simulink model "tcs_VHF_model_free"  (R2022b)
settings: Solver=FixedStepAuto  StartTime=0.0  StopTime=6.5  RelTol=1e-3
PreLoadFcn:
  | run('control_bus.m')
model workspace (MAT data in the model file):
  Tmax = 1000
  re = 0.284
libraries: simulink x4, Solver_SF x1
CloseFcn:
  | clear control_info_bus
settings Model: Creator=henri  LastModifiedBy=Henrique Mesquita
settings DebuggingCC: UnconnectedInputMsg=warning  UnconnectedOutputMsg=warning  UnconnectedLineMsg=warning
settings ModelReferenceCC: EnableRefExpFcnMdlSchedulingChecks=on
settings RTWCC: DLArmComputeVersion=19.05

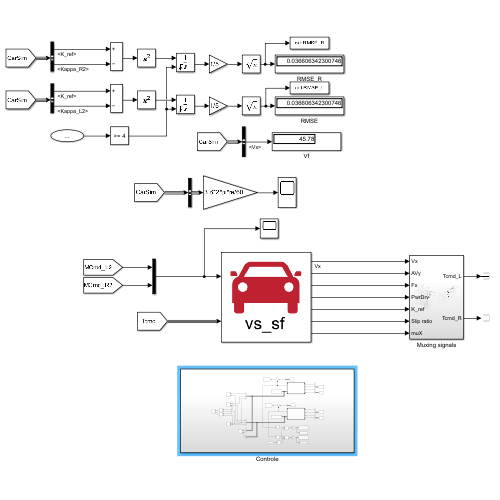
[thumbnail: Simulink's stored preview of the top-level diagram]
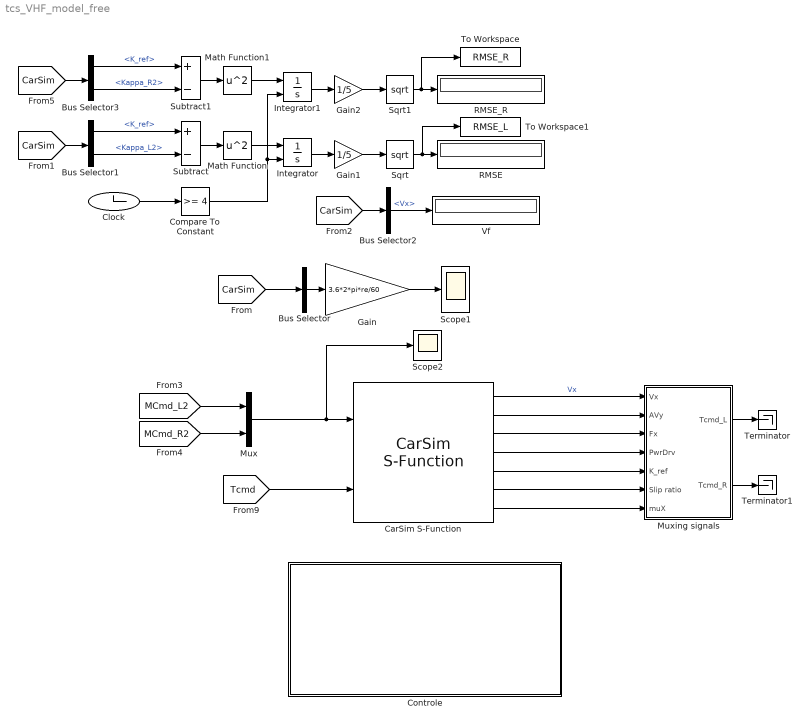
== system tcs_VHF_model_free ==
  Bus Selector : BusSelector  OutputSignals=AVy_L1,AVy_R1,AVy_L2,AVy_R2  OutputAsBus=on
  Bus Selector1 : BusSelector  OutputSignals=K_ref,Kappa_L2
  Bus Selector2 : BusSelector  OutputSignals=Vx
  Bus Selector3 : BusSelector  OutputSignals=K_ref,Kappa_R2
  CarSim S-Function : Solver_SF/CarSim S-Function  Priority=1  SIMFILE=simfile.sim  Run_RTs=off  vs_state_ind=Run  StopMode_ind=Vehicle Model
  Clock : Clock
  Compare To Constant : simulink/Logic and Bit Operations/Compare To Constant  relop=>=  const=4  OutDataTypeStr=boolean
  Controle : Subsystem
  Gain : Gain  Gain=3.6*2*pi*re/60
  Gain1 : Gain  Gain=1/5
  Gain2 : Gain  Gain=1/5
  Integrator : Integrator  ExternalReset=rising
  Integrator1 : Integrator  ExternalReset=rising
  Math Function : Math  Operator=square
  Math Function1 : Math  Operator=square
  Mux : Mux  Inputs=2
  Muxing signals : Subsystem
  RMSE : Display
  RMSE_R : Display
  Scope1 : Scope
  Scope2 : Scope
  Sqrt : Sqrt
  Sqrt1 : Sqrt
  Subtract : Sum  Inputs=+-
  Subtract1 : Sum  Inputs=+-
  Terminator : Terminator
  Terminator1 : Terminator
  To Workspace : ToWorkspace  VariableName=RMSE_R  SampleTime=-1
      settings: MaxDataPoints=1  Save2DSignal=2-D array (concatenate along first dimension)
  To Workspace1 : ToWorkspace  VariableName=RMSE_L  SampleTime=-1
      settings: MaxDataPoints=1  Save2DSignal=2-D array (concatenate along first dimension)
  Vf : Display
  wires:
  Mux/1 -> Scope2/1, CarSim S-Function/1
  [CarSim] -> Bus Selector/1
  Bus Selector/1 -> Gain/1
  [MCmd_R2] -> Mux/2
  [MCmd_L2] -> Mux/1
  [Tcmd] -> CarSim S-Function/2
  CarSim S-Function/1 -> Muxing signals/1(Vx)  "Vx"
  CarSim S-Function/2 -> Muxing signals/2(AVy)
  CarSim S-Function/3 -> Muxing signals/3(Fx)
  CarSim S-Function/4 -> Muxing signals/4(PwrDrv)
  CarSim S-Function/6 -> Muxing signals/6(Slip ratio)
  Muxing signals/2(Tcmd_R) -> Terminator1/1
  Muxing signals/1(Tcmd_L) -> Terminator/1
  CarSim S-Function/5 -> Muxing signals/5(K_ref)
  CarSim S-Function/7 -> Muxing signals/7(muX)
  Gain/1 -> Scope1/1
  [CarSim] -> Bus Selector1/1
  Bus Selector1/2 -> Subtract/2  "<Kappa_L2>"
  Bus Selector1/1 -> Subtract/1  "<K_ref>"
  Integrator/1 -> Gain1/1
  Gain1/1 -> Sqrt/1
  Subtract/1 -> Math Function/1
  Math Function/1 -> Integrator/1
  Sqrt/1 -> To Workspace1/1, RMSE/1
  [CarSim] -> Bus Selector2/1
  Bus Selector2/1 -> Vf/1  "<Vx>"
  Sqrt1/1 -> To Workspace/1, RMSE_R/1
  Integrator1/1 -> Gain2/1
  Gain2/1 -> Sqrt1/1
  Subtract1/1 -> Math Function1/1
  Bus Selector3/1 -> Subtract1/1  "<K_ref>"
  [CarSim] -> Bus Selector3/1
  Math Function1/1 -> Integrator1/1
  Bus Selector3/2 -> Subtract1/2  "<Kappa_R2>"
  Clock/1 -> Compare To Constant/1
  Compare To Constant/1 -> Integrator/2, Integrator1/2

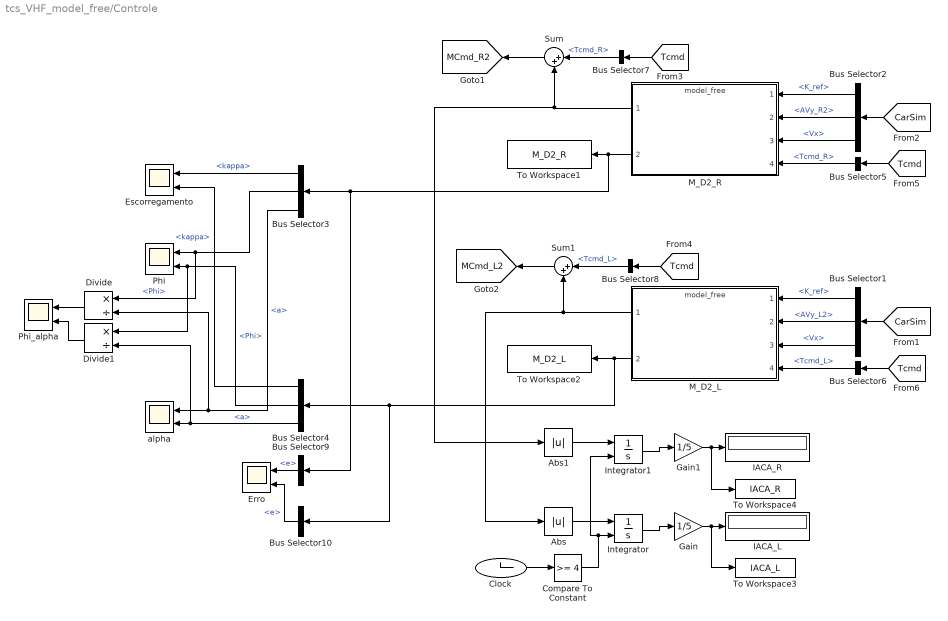
== system tcs_VHF_model_free/Controle ==
  Abs : Abs  SaturateOnIntegerOverflow=off
  Abs1 : Abs  SaturateOnIntegerOverflow=off
  Bus Selector1 : BusSelector  OutputSignals=K_ref,AVy_L2,Vx
  Bus Selector10 : BusSelector  OutputSignals=e
  Bus Selector2 : BusSelector  OutputSignals=K_ref,AVy_R2,Vx
  Bus Selector3 : BusSelector  OutputSignals=kappa,Phi,a
  Bus Selector4 : BusSelector  OutputSignals=kappa,Phi,a
  Bus Selector5 : BusSelector  OutputSignals=Tcmd_R
  Bus Selector6 : BusSelector  OutputSignals=Tcmd_L
  Bus Selector7 : BusSelector  OutputSignals=Tcmd_R
  Bus Selector8 : BusSelector  OutputSignals=Tcmd_L
  Bus Selector9 : BusSelector  OutputSignals=e
  Clock : Clock
  Compare To Constant : simulink/Logic and Bit Operations/Compare To Constant  relop=>=  const=4  OutDataTypeStr=boolean
  Divide : Product  Inputs=*/
  Divide1 : Product  Inputs=*/
  Erro : Scope  NumInputPorts=2
  "Escorregamento " : Scope  NumInputPorts=2
  Gain : Gain  Gain=1/5
  Gain1 : Gain  Gain=1/5
  IACA_L : Display
  IACA_R : Display
  Integrator : Integrator  ExternalReset=rising
  Integrator1 : Integrator  ExternalReset=rising
  M_D2_L : ModelReference  ModelNameDialog=model_free.slx  SimulationMode=Normal  ModelReferenceVersion=4.1
  M_D2_R : ModelReference  ModelNameDialog=model_free.slx  SimulationMode=Normal  ModelReferenceVersion=4.1
  Phi : Scope  NumInputPorts=2
  Phi_alpha : Scope  NumInputPorts=2
  Sum : Sum  Inputs=|++
  Sum1 : Sum  Inputs=|++
  To Workspace1 : ToWorkspace  VariableName=M_D2_R  SaveFormat=Timeseries  SampleTime=-1
  To Workspace2 : ToWorkspace  VariableName=M_D2_L  SaveFormat=Timeseries  SampleTime=-1
  To Workspace3 : ToWorkspace  VariableName=IACA_L  SampleTime=-1
      settings: MaxDataPoints=1  Save2DSignal=2-D array (concatenate along first dimension)
  To Workspace4 : ToWorkspace  VariableName=IACA_R  SampleTime=-1
      settings: MaxDataPoints=1  Save2DSignal=2-D array (concatenate along first dimension)
  alpha : Scope  NumInputPorts=2
  tag scope: MCmd_L2=global, MCmd_R2=global
  wires:
  Bus Selector4/3 -> Divide1/2, alpha/2  "<a>"
  M_D2_L/2 -> To Workspace2/1, Bus Selector10/1, Bus Selector4/1
  M_D2_R/2 -> To Workspace1/1, Bus Selector9/1, Bus Selector3/1
  [CarSim] -> Bus Selector1/1
  Bus Selector1/2 -> M_D2_L/2  "<AVy_L2>"
  Bus Selector2/2 -> M_D2_R/2  "<AVy_R2>"
  Bus Selector1/3 -> M_D2_L/3  "<Vx>"
  [CarSim] -> Bus Selector2/1
  Bus Selector2/3 -> M_D2_R/3  "<Vx>"
  Bus Selector6/1 -> M_D2_L/4  "<Tcmd_L>"
  Bus Selector4/2 -> Divide1/1, Phi/2  "<Phi>"
  Bus Selector3/2 -> Divide/1, Phi/1  "<Phi>"
  Bus Selector4/1 -> "Escorregamento "/2  "<kappa>"
  M_D2_R/1 -> Abs1/1, Sum/2
  Bus Selector3/1 -> "Escorregamento "/1  "<kappa>"
  [Tcmd] -> Bus Selector6/1
  Bus Selector2/1 -> M_D2_R/1  "<K_ref>"
  Bus Selector1/1 -> M_D2_L/1  "<K_ref>"
  [Tcmd] -> Bus Selector5/1
  Bus Selector3/3 -> Divide/2, alpha/1  "<a>"
  Bus Selector5/1 -> M_D2_R/4  "<Tcmd_R>"
  Sum/1 -> [MCmd_R2]
  [Tcmd] -> Bus Selector7/1
  Bus Selector7/1 -> Sum/1  "<Tcmd_R>"
  Bus Selector8/1 -> Sum1/1  "<Tcmd_L>"
  [Tcmd] -> Bus Selector8/1
  M_D2_L/1 -> Abs/1, Sum1/2
  Sum1/1 -> [MCmd_L2]
  Divide/1 -> Phi_alpha/1
  Divide1/1 -> Phi_alpha/2
  Bus Selector9/1 -> Erro/1  "<e>"
  Bus Selector10/1 -> Erro/2  "<e>"
  Abs/1 -> Integrator/1
  Integrator/1 -> Gain/1
  Gain/1 -> To Workspace3/1, IACA_L/1
  Clock/1 -> Compare To Constant/1
  Compare To Constant/1 -> Integrator/2, Integrator1/2
  Abs1/1 -> Integrator1/1
  Gain1/1 -> To Workspace4/1, IACA_R/1
  Integrator1/1 -> Gain1/1

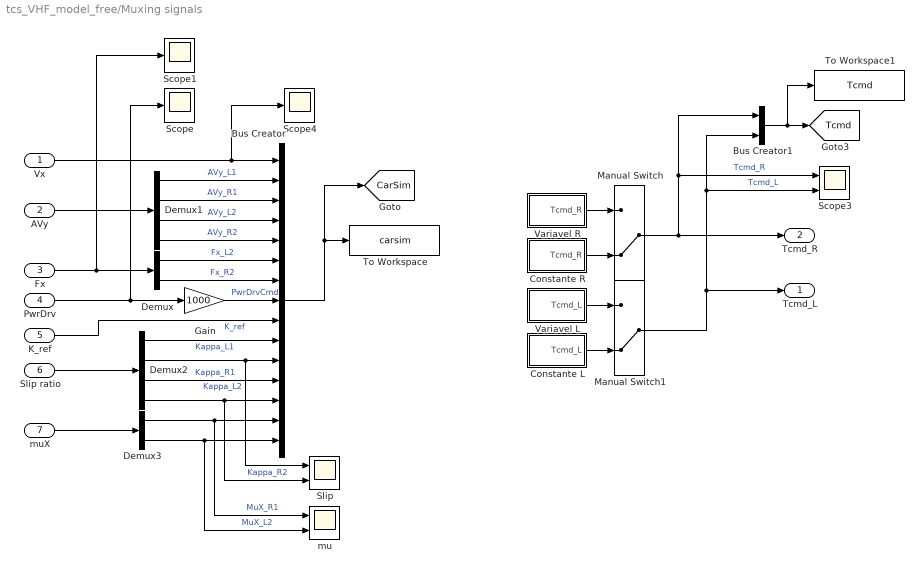
== system tcs_VHF_model_free/Muxing signals ==
  Vx : Inport
  AVy : Inport  Port=2
  Fx : Inport  Port=3
  PwrDrv : Inport  Port=4
  K_ref : Inport  Port=5
  Slip ratio : Inport  Port=6
  muX : Inport  Port=7
  Bus Creator : BusCreator  Inputs=15
  Bus Creator1 : BusCreator  Inputs=2
  Constante L : Subsystem
  Constante R : Subsystem
  Demux : Demux  Outputs=2
  Demux1 : Demux
  Demux2 : Demux
  Demux3 : Demux  Outputs=2
  Gain : Gain  Gain=1000
  Manual Switch : ManualSwitch  CurrentSetting=0
  Manual Switch1 : ManualSwitch  CurrentSetting=0
  Scope : Scope
  Scope1 : Scope
  Scope3 : Scope  NumInputPorts=2
  Scope4 : Scope
  Slip : Scope  NumInputPorts=2
  To Workspace : ToWorkspace  VariableName=carsim  SaveFormat=Timeseries  SampleTime=-1
  To Workspace1 : ToWorkspace  VariableName=Tcmd  SaveFormat=Timeseries  SampleTime=-1
  Variavel L : Subsystem
  Variavel R : Subsystem
  mu : Scope  NumInputPorts=2
  Tcmd_L : Outport
  Tcmd_R : Outport  Port=2
  tag scope: CarSim=global, Tcmd=global
  wires:
  K_ref/1 -> Bus Creator/9  "K_ref"
  Demux1/3 -> Bus Creator/4  "AVy_L2"
  Bus Creator/1 -> [CarSim], To Workspace/1
  Demux/2 -> Bus Creator/7  "Fx_R2"
  Vx/1 -> Scope4/1, Bus Creator/1
  Demux1/1 -> Bus Creator/2  "AVy_L1"
  Demux1/4 -> Bus Creator/5  "AVy_R2"
  PwrDrv/1 -> Gain/1, Scope/1
  Demux/1 -> Bus Creator/6  "Fx_L2"
  Gain/1 -> Bus Creator/8  "PwrDrvCmd"
  Demux1/2 -> Bus Creator/3  "AVy_R1"
  Fx/1 -> Scope1/1, Demux/1
  AVy/1 -> Demux1/1
  Bus Creator1/1 -> To Workspace1/1, [Tcmd]
  Manual Switch/1 -> Bus Creator1/1, Scope3/1, Tcmd_R/1  "Tcmd_R"
  Manual Switch1/1 -> Bus Creator1/2, Scope3/2, Tcmd_L/1  "Tcmd_L"
  Slip ratio/1 -> Demux2/1
  Demux2/1 -> Bus Creator/10  "Kappa_L1"
  Demux2/2 -> Slip/1, Bus Creator/11  "Kappa_L2"
  Demux2/3 -> Bus Creator/12  "Kappa_R1"
  Demux2/4 -> Slip/2, Bus Creator/13  "Kappa_R2"
  Variavel R/1(Tcmd_R) -> Manual Switch/1
  Constante R/1(Tcmd_R) -> Manual Switch/2
  Constante L/1(Tcmd_L) -> Manual Switch1/2
  Variavel L/1(Tcmd_L) -> Manual Switch1/1
  muX/1 -> Demux3/1
  Demux3/1 -> mu/1, Bus Creator/14  "MuX_R1"
  Demux3/2 -> mu/2, Bus Creator/15  "MuX_L2"

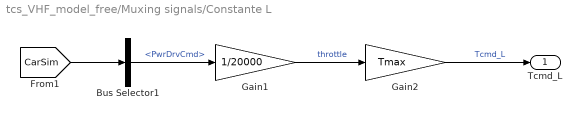
== system tcs_VHF_model_free/Muxing signals/Constante L ==
  Bus Selector1 : BusSelector  OutputSignals=PwrDrvCmd
  Gain1 : Gain  Gain=1/20000
  Gain2 : Gain  Gain=Tmax
  Tcmd_L : Outport
  wires:
  Gain2/1 -> Tcmd_L/1  "Tcmd_L"
  Gain1/1 -> Gain2/1  "throttle"
  [CarSim] -> Bus Selector1/1
  Bus Selector1/1 -> Gain1/1  "<PwrDrvCmd>"

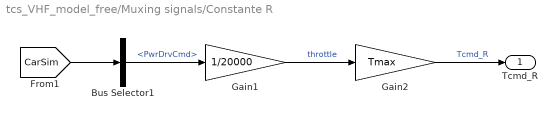
== system tcs_VHF_model_free/Muxing signals/Constante R ==
  Bus Selector1 : BusSelector  OutputSignals=PwrDrvCmd
  Gain1 : Gain  Gain=1/20000
  Gain2 : Gain  Gain=Tmax
  Tcmd_R : Outport
  wires:
  Gain2/1 -> Tcmd_R/1  "Tcmd_R"
  Gain1/1 -> Gain2/1  "throttle"
  [CarSim] -> Bus Selector1/1
  Bus Selector1/1 -> Gain1/1  "<PwrDrvCmd>"

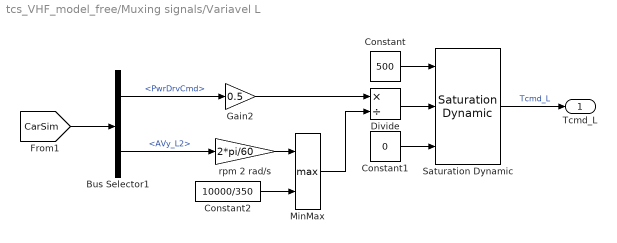
== system tcs_VHF_model_free/Muxing signals/Variavel L ==
  Bus Selector1 : BusSelector  OutputSignals=PwrDrvCmd,AVy_L2
  Constant : Constant  Value=500
  Constant1 : Constant  Value=0
  Constant2 : Constant  Value=10000/350
  Divide : Product  Inputs=*/
  Gain2 : Gain  Gain=0.5
  MinMax : MinMax  Function=max  Inputs=2
  Saturation Dynamic : simulink/Discontinuities/Saturation Dynamic  OutMin=[]  OutMax=[]  OutDataTypeStr=Inherit: Same as second input  OutDataType=fixdt(1, 16)  OutScaling=2^-10  DoSatur=off
  rpm 2 rad/s : Gain  Gain=2*pi/60
  Tcmd_L : Outport
  wires:
  [CarSim] -> Bus Selector1/1
  Bus Selector1/1 -> Gain2/1  "<PwrDrvCmd>"
  Divide/1 -> Saturation Dynamic/2
  Constant1/1 -> Saturation Dynamic/3
  Bus Selector1/2 -> rpm 2 rad/s/1  "<AVy_L2>"
  Gain2/1 -> Divide/1
  Saturation Dynamic/1 -> Tcmd_L/1  "Tcmd_L"
  rpm 2 rad/s/1 -> MinMax/1
  MinMax/1 -> Divide/2
  Constant2/1 -> MinMax/2
  Constant/1 -> Saturation Dynamic/1

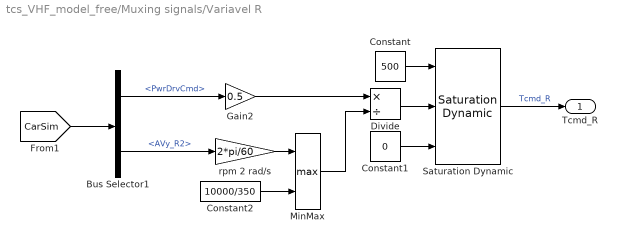
== system tcs_VHF_model_free/Muxing signals/Variavel R ==
  Bus Selector1 : BusSelector  OutputSignals=PwrDrvCmd,AVy_R2
  Constant : Constant  Value=500
  Constant1 : Constant  Value=0
  Constant2 : Constant  Value=10000/350
  Divide : Product  Inputs=*/
  Gain2 : Gain  Gain=0.5
  MinMax : MinMax  Function=max  Inputs=2
  Saturation Dynamic : simulink/Discontinuities/Saturation Dynamic  OutMin=[]  OutMax=[]  OutDataTypeStr=Inherit: Same as second input  OutDataType=fixdt(1, 16)  OutScaling=2^-10  DoSatur=off
  rpm 2 rad/s : Gain  Gain=2*pi/60
  Tcmd_R : Outport
  wires:
  [CarSim] -> Bus Selector1/1
  Bus Selector1/1 -> Gain2/1  "<PwrDrvCmd>"
  Divide/1 -> Saturation Dynamic/2
  Constant1/1 -> Saturation Dynamic/3
  Bus Selector1/2 -> rpm 2 rad/s/1  "<AVy_R2>"
  Constant/1 -> Saturation Dynamic/1
  Gain2/1 -> Divide/1
  Saturation Dynamic/1 -> Tcmd_R/1  "Tcmd_R"
  rpm 2 rad/s/1 -> MinMax/1
  MinMax/1 -> Divide/2
  Constant2/1 -> MinMax/2
